simulink library "jeb"  (Simulink 8.1)
settings: Solver=ode45  StartTime=0.0  StopTime=10.0  RelTol=1e-3
libraries: asr x1, aab x1, adc x1, afrt x1, aro x1, aec x1, aac x1, atc x1, pbv x1, aoc x1
settings Model: Creator=xsellart  LastModifiedBy=AT015555

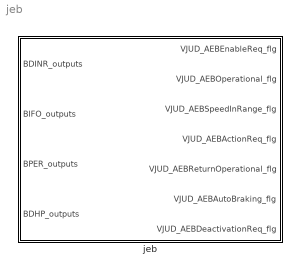
== system jeb ==
  jeb : Subsystem

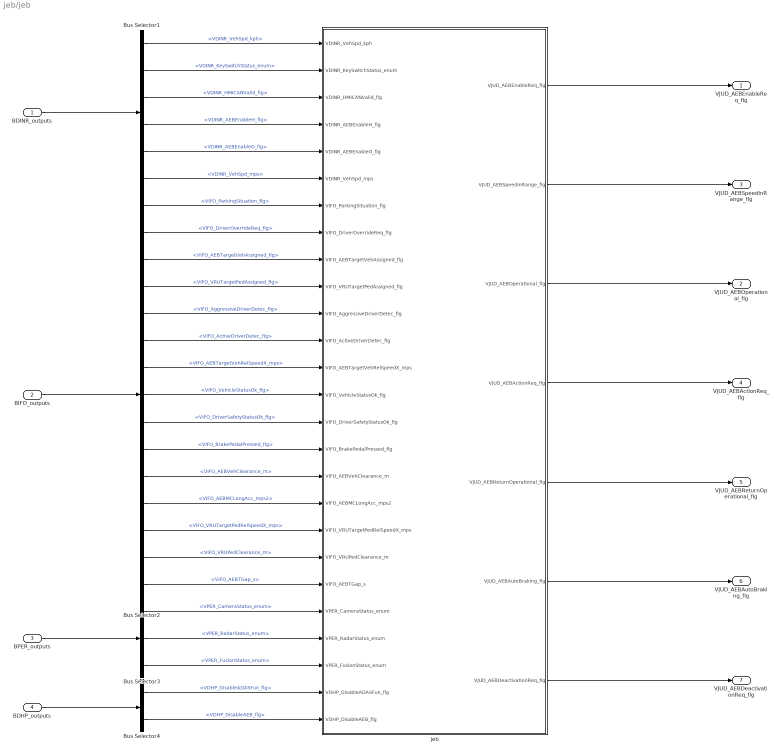
== system jeb/jeb ==
  BDINR_outputs : Inport  OutDataTypeStr=Bus: BDINR_outputs
  BIFO_outputs : Inport  Port=2  OutDataTypeStr=Bus: BIFO_outputs
  BPER_outputs : Inport  Port=3  OutDataTypeStr=Bus: BPER_outputs
  BDHP_outputs : Inport  Port=4  OutDataTypeStr=Bus: BDHP_outputs
  Bus Selector1 : BusSelector  OutputSignals=VDINR_VehSpd_kph,VDINR_KeySwitchStatus_enum,VDINR_HMICANValid_flg,VDINR_AEBEnableH_flg,VDINR_AEBEnableO_flg,VDINR_VehSpd_mps
  Bus Selector2 : BusSelector  OutputSignals=VIFO_ParkingSituation_flg,VIFO_DriverOverrideReq_flg,VIFO_AEBTargetVehAssigned_flg,VIFO_VRUTargetPedAssigned_flg,VIFO_AggressiveDriverDetec_flg,VIFO_ActiveDriverDetec_flg,VIFO_AEBTargetVehRelSpeedX_mps,VIFO_VehicleStatusOk_flg,VIFO_DriverSafetyStatusOk_flg,VIFO_BrakePedalPressed_flg,VIFO_AEBVehClearance_m,VIFO_AEBMCLongAcc_mps2,VIFO_VRUTargetPedRelSpeedX_mps,VIFO_VRUPedClearance_m,VIFO_AEBTGap_s
  Bus Selector3 : BusSelector  OutputSignals=VPER_CameraStatus_enum,VPER_RadarStatus_enum,VPER_FusionStatus_enum
  Bus Selector4 : BusSelector  OutputSignals=VDHP_DisableADASFun_flg,VDHP_DisableAEB_flg
  jeb : Subsystem
  VJUD_AEBEnableReq_flg : Outport
  VJUD_AEBOperational_flg : Outport  Port=2
  VJUD_AEBSpeedInRange_flg : Outport  Port=3
  VJUD_AEBActionReq_flg : Outport  Port=4
  VJUD_AEBReturnOperational_flg : Outport  Port=5
  VJUD_AEBAutoBraking_flg : Outport  Port=6
  VJUD_AEBDeactivationReq_flg : Outport  Port=7
  wires:
  jeb/1(VJUD_AEBEnableReq_flg) -> VJUD_AEBEnableReq_flg/1
  jeb/2(VJUD_AEBSpeedInRange_flg) -> VJUD_AEBSpeedInRange_flg/1
  jeb/3(VJUD_AEBOperational_flg) -> VJUD_AEBOperational_flg/1
  jeb/4(VJUD_AEBActionReq_flg) -> VJUD_AEBActionReq_flg/1
  jeb/6(VJUD_AEBAutoBraking_flg) -> VJUD_AEBAutoBraking_flg/1
  jeb/7(VJUD_AEBDeactivationReq_flg) -> VJUD_AEBDeactivationReq_flg/1
  BDINR_outputs/1 -> Bus Selector1/1
  BIFO_outputs/1 -> Bus Selector2/1
  Bus Selector1/2 -> jeb/2(VDINR_KeySwitchStatus_enum)  "<VDINR_KeySwitchStatus_enum>"
  Bus Selector3/1 -> jeb/22(VPER_CameraStatus_enum)  "<VPER_CameraStatus_enum>"
  Bus Selector1/3 -> jeb/3(VDINR_HMICANValid_flg)  "<VDINR_HMICANValid_flg>"
  Bus Selector1/1 -> jeb/1(VDINR_VehSpd_kph)  "<VDINR_VehSpd_kph>"
  Bus Selector1/5 -> jeb/5(VDINR_AEBEnableO_flg)  "<VDINR_AEBEnableO_flg>"
  Bus Selector2/3 -> jeb/9(VIFO_AEBTargetVehAssigned_flg)  "<VIFO_AEBTargetVehAssigned_flg>"
  Bus Selector2/8 -> jeb/14(VIFO_VehicleStatusOk_flg)  "<VIFO_VehicleStatusOk_flg>"
  Bus Selector2/5 -> jeb/11(VIFO_AggressiveDriverDetec_flg)  "<VIFO_AggressiveDriverDetec_flg>"
  Bus Selector2/9 -> jeb/15(VIFO_DriverSafetyStatusOk_flg)  "<VIFO_DriverSafetyStatusOk_flg>"
  Bus Selector2/2 -> jeb/8(VIFO_DriverOverrideReq_flg)  "<VIFO_DriverOverrideReq_flg>"
  Bus Selector2/7 -> jeb/13(VIFO_AEBTargetVehRelSpeedX_mps)  "<VIFO_AEBTargetVehRelSpeedX_mps>"
  Bus Selector2/6 -> jeb/12(VIFO_ActiveDriverDetec_flg)  "<VIFO_ActiveDriverDetec_flg>"
  Bus Selector2/1 -> jeb/7(VIFO_ParkingSituation_flg)  "<VIFO_ParkingSituation_flg>"
  Bus Selector3/2 -> jeb/23(VPER_RadarStatus_enum)  "<VPER_RadarStatus_enum>"
  Bus Selector3/3 -> jeb/24(VPER_FusionStatus_enum)  "<VPER_FusionStatus_enum>"
  BPER_outputs/1 -> Bus Selector3/1
  Bus Selector4/1 -> jeb/25(VDHP_DisableADASFun_flg)  "<VDHP_DisableADASFun_flg>"
  Bus Selector4/2 -> jeb/26(VDHP_DisableAEB_flg)  "<VDHP_DisableAEB_flg>"
  BDHP_outputs/1 -> Bus Selector4/1
  Bus Selector1/4 -> jeb/4(VDINR_AEBEnableH_flg)  "<VDINR_AEBEnableH_flg>"
  Bus Selector2/10 -> jeb/16(VIFO_BrakePedalPressed_flg)  "<VIFO_BrakePedalPressed_flg>"
  jeb/5(VJUD_AEBReturnOperational_flg) -> VJUD_AEBReturnOperational_flg/1
  Bus Selector2/11 -> jeb/17(VIFO_AEBVehClearance_m)  "<VIFO_AEBVehClearance_m>"
  Bus Selector1/6 -> jeb/6(VDINR_VehSpd_mps)  "<VDINR_VehSpd_mps>"
  Bus Selector2/12 -> jeb/18(VIFO_AEBMCLongAcc_mps2)  "<VIFO_AEBMCLongAcc_mps2>"
  Bus Selector2/13 -> jeb/19(VIFO_VRUTargetPedRelSpeedX_mps)  "<VIFO_VRUTargetPedRelSpeedX_mps>"
  Bus Selector2/4 -> jeb/10(VIFO_VRUTargetPedAssigned_flg)  "<VIFO_VRUTargetPedAssigned_flg>"
  Bus Selector2/14 -> jeb/20(VIFO_VRUPedClearance_m)  "<VIFO_VRUPedClearance_m>"
  Bus Selector2/15 -> jeb/21(VIFO_AEBTGap_s)  "<VIFO_AEBTGap_s>"

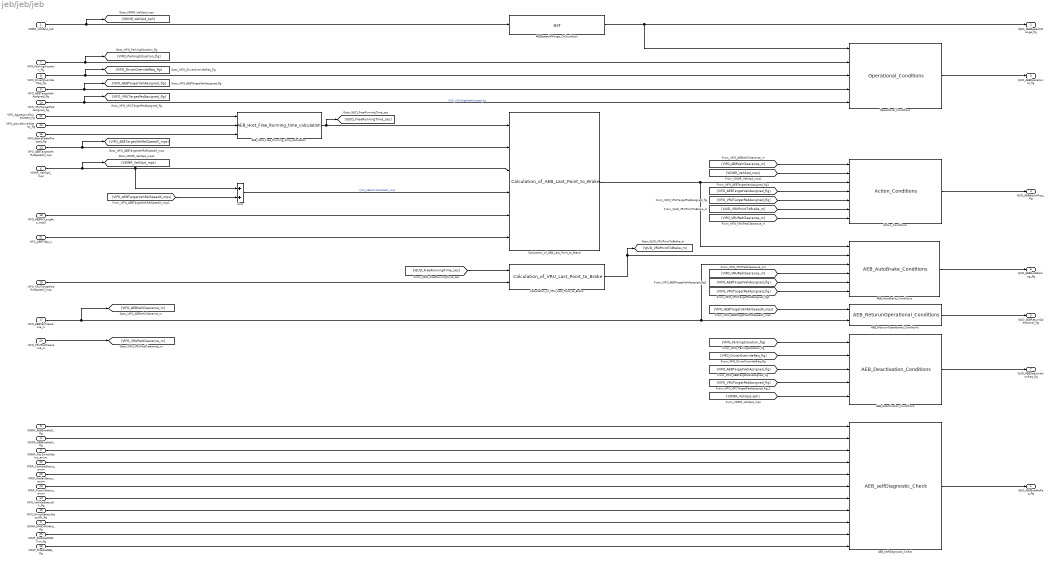
== system jeb/jeb/jeb ==
  VDINR_VehSpd_kph : Inport
  VDINR_KeySwitchStatus_enum : Inport  Port=2
  VDINR_HMICANValid_flg : Inport  Port=3
  VDINR_AEBEnableH_flg : Inport  Port=4
  VDINR_AEBEnableO_flg : Inport  Port=5
  VDINR_VehSpd_mps : Inport  Port=6
  VIFO_ParkingSituation_flg : Inport  Port=7
  VIFO_DriverOverrideReq_flg : Inport  Port=8
  VIFO_AEBTargetVehAssigned_flg : Inport  Port=9
  VIFO_VRUTargetPedAssigned_flg : Inport  Port=10
  VIFO_AggressiveDriverDetec_flg : Inport  Port=11
  VIFO_ActiveDriverDetec_flg : Inport  Port=12
  VIFO_AEBTargetVehRelSpeedX_mps : Inport  Port=13
  VIFO_VehicleStatusOk_flg : Inport  Port=14
  VIFO_DriverSafetyStatusOk_flg : Inport  Port=15
  VIFO_BrakePedalPressed_flg : Inport  Port=16
  VIFO_AEBVehClearance_m : Inport  Port=17
  VIFO_AEBMCLongAcc_mps2 : Inport  Port=18
  VIFO_VRUTargetPedRelSpeedX_mps : Inport  Port=19
  VIFO_VRUPedClearance_m : Inport  Port=20
  VIFO_AEBTGap_s : Inport  Port=21
  VPER_CameraStatus_enum : Inport  Port=22
  VPER_RadarStatus_enum : Inport  Port=23
  VPER_FusionStatus_enum : Inport  Port=24
  VDHP_DisableADASFun_flg : Inport  Port=25
  VDHP_DisableAEB_flg : Inport  Port=26
  AEBSpeedInRange_Caluculation : asr/asr
  AEB_AutoBrake_Conditions : aab/AEB_AutoBrake_Conditions
  AEB_Deactivation_Conditions : adc/AEB_Deactivation_Conditions
  AEB_Host_Free_Running_time_calculation : afrt/AEB_Host_Free_Running_time_calculation
  AEB_ReturunOperational_Conditions : aro/AEB_ReturunOperational_Conditions
  AEB_selfDiagnostic_Check : aec/AEB_selfDiagnostic_Check
  Action_Conditions : aac/Action_Conditions
  Calculation_of_AEB_Last_Point_to_Brake : atc/Calculation_of_AEB_Last_Point_to_Brake
  Calculation_of_VRU_Last_Point_to_Brake : pbv/Calculation_of_VRU_Last_Point_to_Brake
  Operational_Conditions : aoc/Operational_Conditions
  Sum : Sum
  VJUD_AEBEnableReq_flg : Outport
  VJUD_AEBSpeedInRange_flg : Outport  Port=2
  VJUD_AEBOperational_flg : Outport  Port=3
  VJUD_AEBActionReq_flg : Outport  Port=4
  VJUD_AEBReturnOperational_flg : Outport  Port=5
  VJUD_AEBAutoBraking_flg : Outport  Port=6
  VJUD_AEBDeactivationReq_flg : Outport  Port=7
  wires:
  VIFO_ActiveDriverDetec_flg/1 -> AEB_Host_Free_Running_time_calculation/2
  VIFO_AggressiveDriverDetec_flg/1 -> AEB_Host_Free_Running_time_calculation/1
  VIFO_DriverOverrideReq_flg/1 -> [VIFO_DriverOverrideReq_flg], Operational_Conditions/3
  VIFO_ParkingSituation_flg/1 -> [VIFO_ParkingSituation_flg], Operational_Conditions/2
  AEBSpeedInRange_Caluculation/1 -> Operational_Conditions/1, VJUD_AEBSpeedInRange_flg/1
  [VIFO_DriverOverrideReq_flg] -> AEB_Deactivation_Conditions/2
  [VIFO_ParkingSituation_flg] -> AEB_Deactivation_Conditions/1
  [VIFO_AEBTargetVehAssigned_flg] -> AEB_Deactivation_Conditions/3
  Action_Conditions/1 -> VJUD_AEBActionReq_flg/1
  Operational_Conditions/1 -> VJUD_AEBOperational_flg/1
  AEB_AutoBrake_Conditions/1 -> VJUD_AEBAutoBraking_flg/1
  AEB_Deactivation_Conditions/1 -> VJUD_AEBDeactivationReq_flg/1
  AEB_selfDiagnostic_Check/1 -> VJUD_AEBEnableReq_flg/1
  VDINR_AEBEnableO_flg/1 -> AEB_selfDiagnostic_Check/1
  VDINR_AEBEnableH_flg/1 -> AEB_selfDiagnostic_Check/2
  VPER_RadarStatus_enum/1 -> AEB_selfDiagnostic_Check/5
  VIFO_DriverSafetyStatusOk_flg/1 -> AEB_selfDiagnostic_Check/8
  VDINR_HMICANValid_flg/1 -> AEB_selfDiagnostic_Check/9
  VPER_FusionStatus_enum/1 -> AEB_selfDiagnostic_Check/6
  VPER_CameraStatus_enum/1 -> AEB_selfDiagnostic_Check/4
  VIFO_VehicleStatusOk_flg/1 -> AEB_selfDiagnostic_Check/7
  VDINR_KeySwitchStatus_enum/1 -> AEB_selfDiagnostic_Check/3
  VDINR_VehSpd_kph/1 -> [VDINR_VehSpd_kph], AEBSpeedInRange_Caluculation/1
  VIFO_BrakePedalPressed_flg/1 -> AEB_Host_Free_Running_time_calculation/3
  VDHP_DisableADASFun_flg/1 -> AEB_selfDiagnostic_Check/10
  VDHP_DisableAEB_flg/1 -> AEB_selfDiagnostic_Check/11
  [VIFO_AEBTargetVehAssigned_flg] -> Action_Conditions/4
  VIFO_AEBTargetVehAssigned_flg/1 -> [VIFO_AEBTargetVehAssigned_flg], Operational_Conditions/4
  VIFO_AEBTargetVehRelSpeedX_mps/1 -> [VIFO_AEBTargetVehRelSpeedX_mps], Calculation_of_AEB_Last_Point_to_Brake/2
  [VDINR_VehSpd_kph] -> AEB_Deactivation_Conditions/5
  AEB_ReturunOperational_Conditions/1 -> VJUD_AEBReturnOperational_flg/1
  VIFO_AEBVehClearance_m/1 -> [VIFO_AEBVehClearance_m], AEB_AutoBrake_Conditions/3, AEB_ReturunOperational_Conditions/2
  Calculation_of_AEB_Last_Point_to_Brake/1 -> AEB_AutoBrake_Conditions/1, Action_Conditions/3
  [VIFO_AEBTargetVehRelSpeedX_mps] -> AEB_ReturunOperational_Conditions/1
  [VIFO_AEBVehClearance_m] -> Action_Conditions/1
  VDINR_VehSpd_mps/1 -> Sum/1, Calculation_of_AEB_Last_Point_to_Brake/3, [VDINR_VehSpd_mps]
  VIFO_AEBMCLongAcc_mps2/1 -> Calculation_of_AEB_Last_Point_to_Brake/5
  [VIFO_AEBTargetVehRelSpeedX_mps] -> Sum/2
  Sum/1 -> Calculation_of_AEB_Last_Point_to_Brake/4  "VJUD_AEBMCVehAbsSpdX_mps"
  [VDINR_VehSpd_mps] -> Action_Conditions/2
  AEB_Host_Free_Running_time_calculation/1 -> Calculation_of_AEB_Last_Point_to_Brake/1, [VJUD_FreeRunningTime_sec]
  [VJUD_FreeRunningTime_sec] -> Calculation_of_VRU_Last_Point_to_Brake/1
  VIFO_VRUTargetPedRelSpeedX_mps/1 -> Calculation_of_VRU_Last_Point_to_Brake/2
  VIFO_VRUTargetPedAssigned_flg/1 -> [VIFO_VRUTargetPedAssigned_flg], Operational_Conditions/5  "VIFO_VRUTargetPedAssigned_flg"
  [VIFO_VRUTargetPedAssigned_flg] -> Action_Conditions/5
  [VIFO_VRUTargetPedAssigned_flg] -> AEB_Deactivation_Conditions/4
  VIFO_VRUPedClearance_m/1 -> [VIFO_VRUPedClearance_m]
  [VIFO_VRUPedClearance_m] -> Action_Conditions/7
  [VJUD_VRUPointToBrake_m] -> Action_Conditions/6
  Calculation_of_VRU_Last_Point_to_Brake/1 -> [VJUD_VRUPointToBrake_m], AEB_AutoBrake_Conditions/2
  [VIFO_VRUPedClearance_m] -> AEB_AutoBrake_Conditions/4
  VIFO_AEBTGap_s/1 -> Calculation_of_AEB_Last_Point_to_Brake/6
  [VIFO_AEBTargetVehAssigned_flg] -> AEB_AutoBrake_Conditions/5
  [VIFO_VRUTargetPedAssigned_flg] -> AEB_AutoBrake_Conditions/6
